simulink model "gear_ctrl"  (R2021b)
settings: Solver=VariableStepAuto  StartTime=0.0  StopTime=inf  RelTol=1e-3
settings Model: Creator=Lenovo  LastModifiedBy=Lenovo

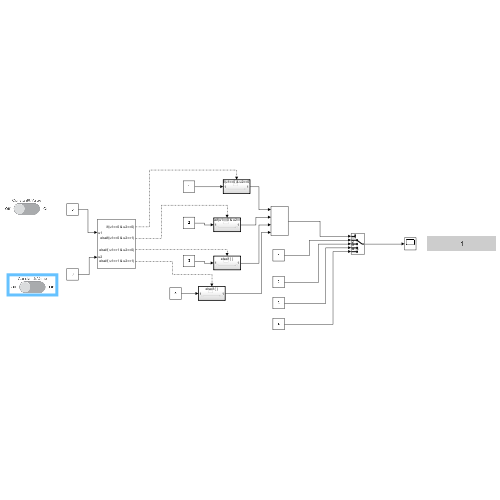
[thumbnail: Simulink's stored preview of the top-level diagram]
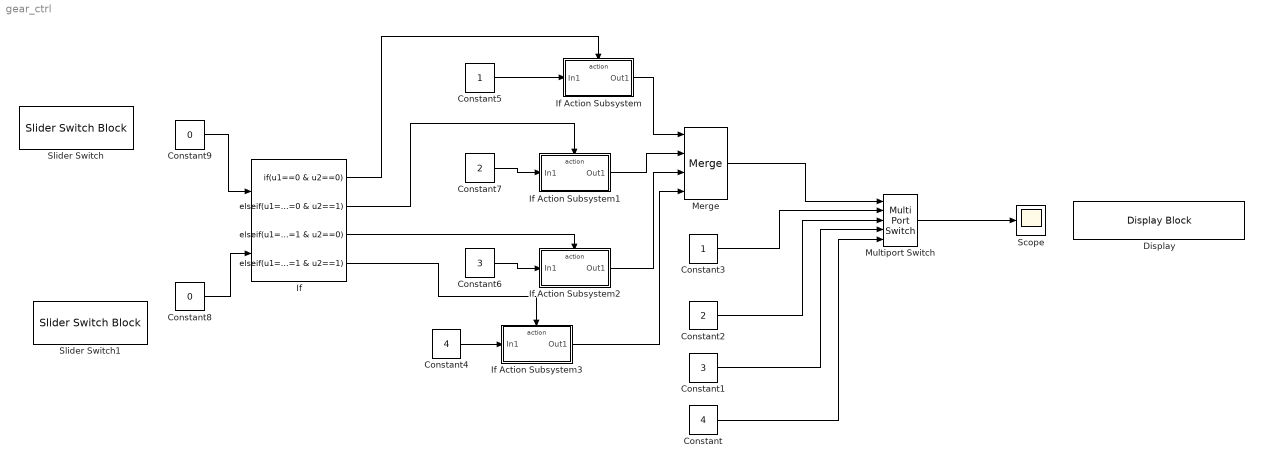
== system gear_ctrl ==
  Constant : Constant  Value=4
  Constant1 : Constant  Value=3
  Constant2 : Constant  Value=2
  Constant3 : Constant
  Constant4 : Constant  Value=4
  Constant5 : Constant
  Constant6 : Constant  Value=3
  Constant7 : Constant  Value=2
  Constant8 : Constant  Value=0
  Constant9 : Constant  Value=0
  Display : DisplayBlock  LabelPosition=Hide  Format=short  Transparency=1
  If : If  NumInputs=2  IfExpression=u1==0 & u2==0  ElseIfExpressions=u1==0 & u2==1, u1==1 & u2==0, u1==1 & u2==1  ShowElse=off
  If Action Subsystem : Subsystem  TreatAsAtomicUnit=on
  If Action Subsystem1 : Subsystem  TreatAsAtomicUnit=on
  If Action Subsystem2 : Subsystem  TreatAsAtomicUnit=on
  If Action Subsystem3 : Subsystem  TreatAsAtomicUnit=on
  Merge : Merge  Inputs=4
  Multiport Switch : MultiPortSwitch  Inputs=4  DiagnosticForDefault=None
  Scope : Scope
  Slider Switch : SliderSwitchBlock
      settings: Values={{'Off', 'On'}, [0 1]}
  Slider Switch1 : SliderSwitchBlock
      settings: Values={{'Off', 'On'}, [0 1]}
  wires:
  Constant9/1 -> If/1
  If/1 -> If Action Subsystem/Action
  If/2 -> If Action Subsystem1/Action
  If/3 -> If Action Subsystem2/Action
  If/4 -> If Action Subsystem3/Action
  Constant4/1 -> If Action Subsystem3/1(In1)
  Constant6/1 -> If Action Subsystem2/1(In1)
  Constant7/1 -> If Action Subsystem1/1(In1)
  Constant5/1 -> If Action Subsystem/1(In1)
  If Action Subsystem/1(Out1) -> Merge/1
  If Action Subsystem1/1(Out1) -> Merge/2
  If Action Subsystem2/1(Out1) -> Merge/3
  If Action Subsystem3/1(Out1) -> Merge/4
  Merge/1 -> Multiport Switch/1
  Constant3/1 -> Multiport Switch/2
  Constant2/1 -> Multiport Switch/3
  Constant1/1 -> Multiport Switch/4
  Constant/1 -> Multiport Switch/5
  Multiport Switch/1 -> Scope/1
  Constant8/1 -> If/2

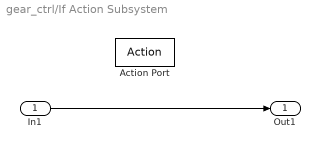
== system gear_ctrl/If Action Subsystem ==
  In1 : Inport
  Action Port : ActionPort  ActionPortLabel=if(u1==0 & u2==0)
  Out1 : Outport
  wires:
  In1/1 -> Out1/1

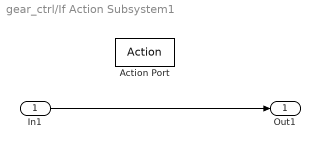
== system gear_ctrl/If Action Subsystem1 ==
  In1 : Inport
  Action Port : ActionPort  ActionPortLabel=elseif(u1==0 & u2==1)
  Out1 : Outport
  wires:
  In1/1 -> Out1/1

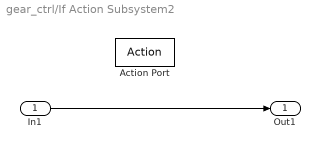
== system gear_ctrl/If Action Subsystem2 ==
  In1 : Inport
  Action Port : ActionPort  ActionPortLabel=elseif( u1==1 & u2==0)
  Out1 : Outport
  wires:
  In1/1 -> Out1/1

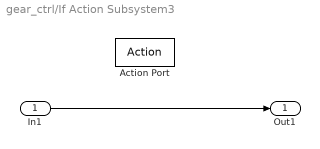
== system gear_ctrl/If Action Subsystem3 ==
  In1 : Inport
  Action Port : ActionPort  ActionPortLabel=elseif( u1==1 & u2==1)
  Out1 : Outport
  wires:
  In1/1 -> Out1/1
